simulink model "moresimilartoopenrocket"  (R2019a)
settings: Solver=ode4  StartTime=0.0  StopTime=6  FixedStep=0.0001  RelTol=1e-3
InitFcn:
  | HeightAboveSeaLevel = 5.4419142084;
  | Temperature = 288.15;
  | Pressure = 	101325;
  | 
  | GustStart = 2.5;
  | GustLength = [100, 100, 100];
  | GuestAmplitude = [ 2.5, -2.5,  1];
  | 
  | ShearSpeed = 10;
  | ShearDirection = 180;
values from neighbouring files (symbols this model uses):
  cg = temp(4)    [NonlinearStateEstimationForActuatorDelay.m]
  F = eye(6)    [MEKFAttitudeOnly.m]
  I = reshape(x(1:9), [3 3])    [AdaptiveLQR.m]    (also in MEKF.m = diag([0.08 0.08 0.002]); MEKFAttitudeOnly.m = diag([0.08 0.08 0.002]); MEKF_old.m = diag([0.08 0.08 0.002]); NonlinearStateEstimationForActuatorDelay.m = diag([Ixx, Ixx, Izz]))
  mass = 1.0565    [ImpactVelocityNotParallelMatlab.m]    (also in NonlinearStateEstimationForActuatorDelay.m = temp(1); OneDLanding.m; RunImpactVelocityParforCompiled.m; Tracker.m = 1.0616753546)
  q = x(13:16)    [AdaptiveLQR.m]    (also in MEKF.m = nominal_state(4:7); MEKFAttitudeOnly.m = [1 0 0 0]; MEKF_old.m = nominal_state(4:7); NonlinearStateEstimationForActuatorDelay.m = x(4:7))
  r = sym('r', [3 1])    [StateSpaceController.m]    (also in TimeDelayCompensationElevator.m = [0;0]; Tracker.m = [0; 0; -(rocket_length - Average_cg)])
undefined symbols (not defined in the file or in its folder): e0_0, e1_0, e2_0, e3_0, Earth, Light, MIL, WGS84
libraries: aerolibutil x5, aerolibwind2 x3, aerolibasang x2, simulink x2, aerolibatmos2 x1, aerolibbdyn x1, simulink_extras x1, aerolibtransform2 x1, sharedtransform x1
settings Model: Creator=rag  LastModifiedBy=rag

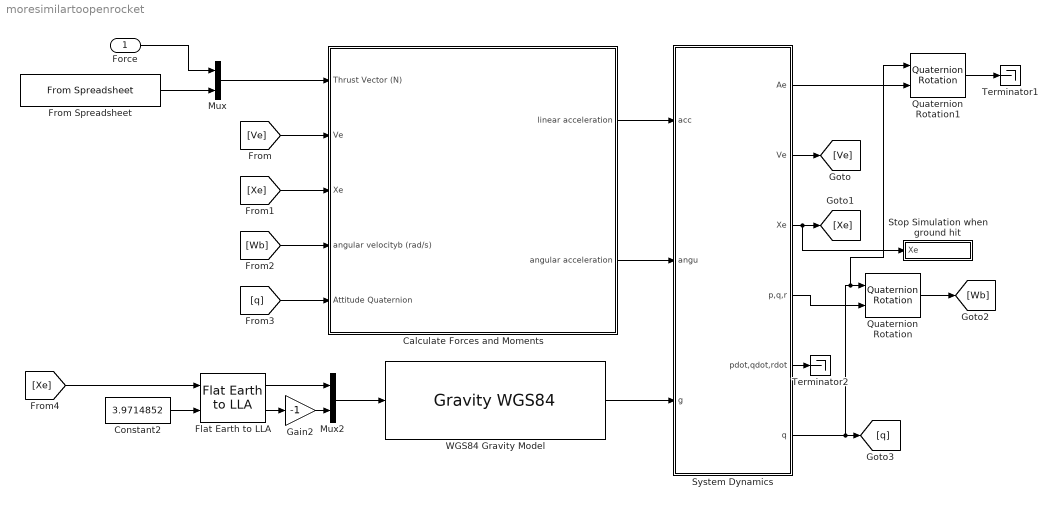
== system moresimilartoopenrocket ==
  Force : Inport  PortDimensions=2
  Calculate Forces and Moments : Subsystem
  Constant2 : Constant  Value=3.9714852
  Flat Earth to LLA : aerolibtransform2/Flat Earth to LLA  units=Metric (MKS)  ptype=Earth (WGS84)  F=1/298.257223563  R=6378137  LL0=[21.318358277648 -157.9232805920725]  psi=052
  From Spreadsheet : FromSpreadsheet  FileName=F10_Thrust.xls  ExtrapolationBeforeFirstDataPoint=Hold first value  ExtrapolationAfterLastDataPoint=Hold last value
  Gain2 : Gain  Gain=-1
  Mux : Mux  Inputs=2
  Mux2 : Mux  Inputs=2
  Quaternion Rotation : aerolibutil/Quaternion Rotation
  Quaternion Rotation1 : aerolibutil/Quaternion Rotation
  Stop Simulation when ground hit : Subsystem
  System Dynamics : Subsystem
  Terminator1 : Terminator
  Terminator2 : Terminator
  "WGS84 Gravity Model  " : GravityWGS84
  wires:
  Calculate Forces and Moments/2(angular acceleration) -> System Dynamics/2(angu)
  Mux/1 -> Calculate Forces and Moments/1(Thrust Vector (N))
  [Ve] -> Calculate Forces and Moments/2(Ve)
  [Xe] -> Calculate Forces and Moments/3(Xe)
  System Dynamics/3(Xe) -> Stop Simulation when ground hit/1(Xe), [Xe]
  Force/1 -> Mux/1
  From Spreadsheet/1 -> Mux/2
  Calculate Forces and Moments/1(linear acceleration) -> System Dynamics/1(acc)
  System Dynamics/2(Ve) -> [Ve]
  [Wb] -> Calculate Forces and Moments/4(angular velocityb (rad/s))
  [q] -> Calculate Forces and Moments/5(Attitude Quaternion)
  System Dynamics/5(pdot,qdot,rdot) -> Terminator2/1
  System Dynamics/6(q) -> [q], Quaternion Rotation1/1, Quaternion Rotation/1
  Constant2/1 -> Flat Earth to LLA/2
  [Xe] -> Flat Earth to LLA/1
  Flat Earth to LLA/1 -> Mux2/1
  Flat Earth to LLA/2 -> Gain2/1
  Mux2/1 -> "WGS84 Gravity Model  "/1
  Gain2/1 -> Mux2/2
  "WGS84 Gravity Model  "/1 -> System Dynamics/3(g)
  Quaternion Rotation/1 -> [Wb]
  System Dynamics/4(p,q,r) -> Quaternion Rotation/2
  Quaternion Rotation1/1 -> Terminator1/1
  System Dynamics/1(Ae) -> Quaternion Rotation1/2

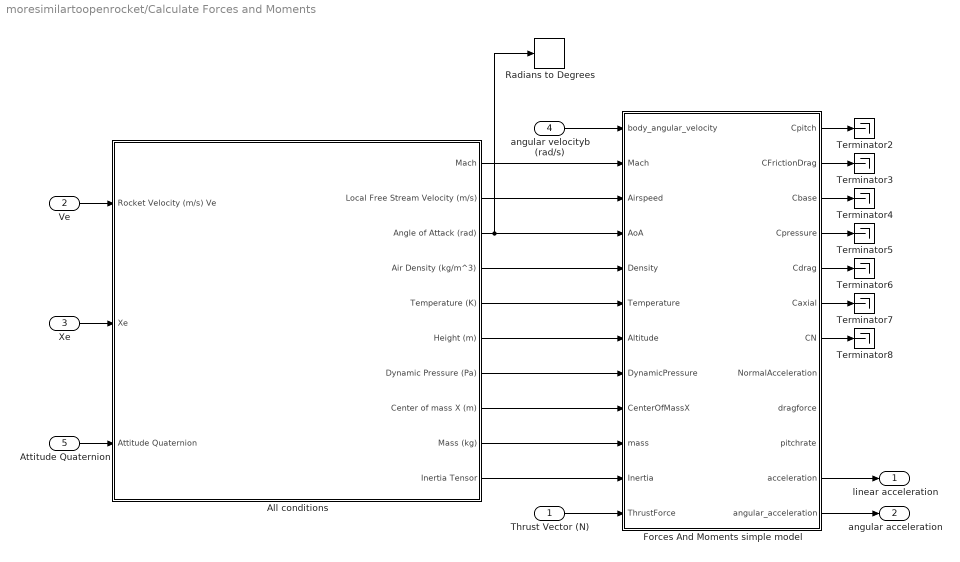
== system moresimilartoopenrocket/Calculate Forces and Moments ==
  Thrust Vector (N) : Inport
  Ve : Inport  Port=2
  Xe : Inport  Port=3
  angular velocityb (rad/s) : Inport  Port=4
  Attitude Quaternion : Inport  Port=5
  All conditions : Subsystem
  Forces And Moments simple model : MATLAB Function  TreatAsAtomicUnit=on
  Radians to Degrees : simulink_extras/Transformations/Radians to Degrees
  Terminator{2..8} (7 alike) : Terminator
  linear acceleration : Outport
  angular acceleration : Outport  Port=2
  wires:
  Forces And Moments simple model/4(Cpressure) -> Terminator5/1
  Xe/1 -> All conditions/2(Xe)
  Attitude Quaternion/1 -> All conditions/3(Attitude Quaternion)
  Forces And Moments simple model/1(Cpitch) -> Terminator2/1
  Forces And Moments simple model/3(Cbase) -> Terminator4/1
  Forces And Moments simple model/5(Cdrag) -> Terminator6/1
  Forces And Moments simple model/2(CFrictionDrag) -> Terminator3/1
  Forces And Moments simple model/6(Caxial) -> Terminator7/1
  Ve/1 -> All conditions/1(Rocket Velocity (m/s) Ve)
  Forces And Moments simple model/7(CN) -> Terminator8/1
  Forces And Moments simple model/12(angular_acceleration) -> angular acceleration/1
  Forces And Moments simple model/11(acceleration) -> linear acceleration/1
  All conditions/1(Mach) -> Forces And Moments simple model/2(Mach)
  All conditions/2(Local Free Stream Velocity (m/s)) -> Forces And Moments simple model/3(Airspeed)
  All conditions/4(Air Density (kg/m^3)) -> Forces And Moments simple model/5(Density)
  All conditions/3(Angle of Attack (rad)) -> Radians to Degrees/1, Forces And Moments simple model/4(AoA)
  All conditions/5(Temperature (K)) -> Forces And Moments simple model/6(Temperature)
  All conditions/7(Dynamic Pressure (Pa)) -> Forces And Moments simple model/8(DynamicPressure)
  All conditions/8(Center of mass X (m)) -> Forces And Moments simple model/9(CenterOfMassX)
  All conditions/6(Height (m)) -> Forces And Moments simple model/7(Altitude)
  All conditions/9(Mass (kg)) -> Forces And Moments simple model/10(mass)
  All conditions/10(Inertia Tensor) -> Forces And Moments simple model/11(Inertia)
  Thrust Vector (N)/1 -> Forces And Moments simple model/12(ThrustForce)
  angular velocityb (rad/s)/1 -> Forces And Moments simple model/1(body_angular_velocity)

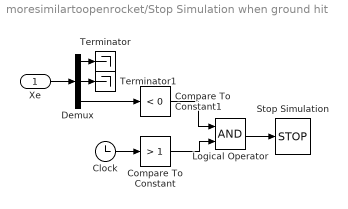
== system moresimilartoopenrocket/Stop Simulation when ground hit ==
  Xe : Inport
  Clock : Clock
  Compare To Constant : simulink/Logic and Bit Operations/Compare To Constant  relop=>  const=1  OutDataTypeStr=boolean
  Compare To Constant1 : simulink/Logic and Bit Operations/Compare To Constant  relop=<  const=0  OutDataTypeStr=boolean
  Demux : Demux  Outputs=3
  Logical Operator : Logic  AllPortsSameDT=off  OutDataTypeStr=boolean
  Stop Simulation : Stop
  Terminator : Terminator
  Terminator1 : Terminator
  wires:
  Logical Operator/1 -> Stop Simulation/1
  Compare To Constant/1 -> Logical Operator/2
  Clock/1 -> Compare To Constant/1
  Compare To Constant1/1 -> Logical Operator/1
  Xe/1 -> Demux/1
  Demux/1 -> Terminator/1
  Demux/2 -> Terminator1/1
  Demux/3 -> Compare To Constant1/1

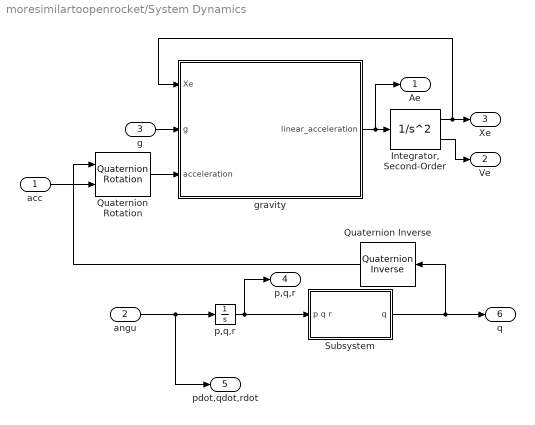
== system moresimilartoopenrocket/System Dynamics ==
  acc : Inport  Unit=N*m  PortDimensions=3
  angu : Inport  Port=2  PortDimensions=3
  g : Inport  Port=3
  "Integrator, Second-Order" : SecondOrderIntegrator
  Quaternion Inverse : aerolibutil/Quaternion Inverse
      settings: SourceProductName=Aerospace Blockset
  Quaternion Rotation : aerolibutil/Quaternion Rotation
  Subsystem : Subsystem
  gravity : MATLAB Function  TreatAsAtomicUnit=on
  "p,q,r " : Integrator
  Ae : Outport  Unit=m/s^2
  Ve : Outport  Port=2  Unit=m/s
  Xe : Outport  Port=3  Unit=m
  p,q,r : Outport  Port=4  Unit=rad/s
  pdot,qdot,rdot : Outport  Port=5  Unit=rad/s^2
  q : Outport  Port=6  Unit=1
  wires:
  "p,q,r "/1 -> p,q,r/1, Subsystem/1(p q r)
  angu/1 -> pdot,qdot,rdot/1, "p,q,r "/1
  acc/1 -> Quaternion Rotation/2
  Subsystem/1(q) -> Quaternion Inverse/1, q/1
  "Integrator, Second-Order"/1 -> Xe/1, gravity/1(Xe)
  "Integrator, Second-Order"/2 -> Ve/1
  Quaternion Rotation/1 -> gravity/3(acceleration)
  gravity/1(linear_acceleration) -> Ae/1, "Integrator, Second-Order"/1
  g/1 -> gravity/2(g)
  Quaternion Inverse/1 -> Quaternion Rotation/1

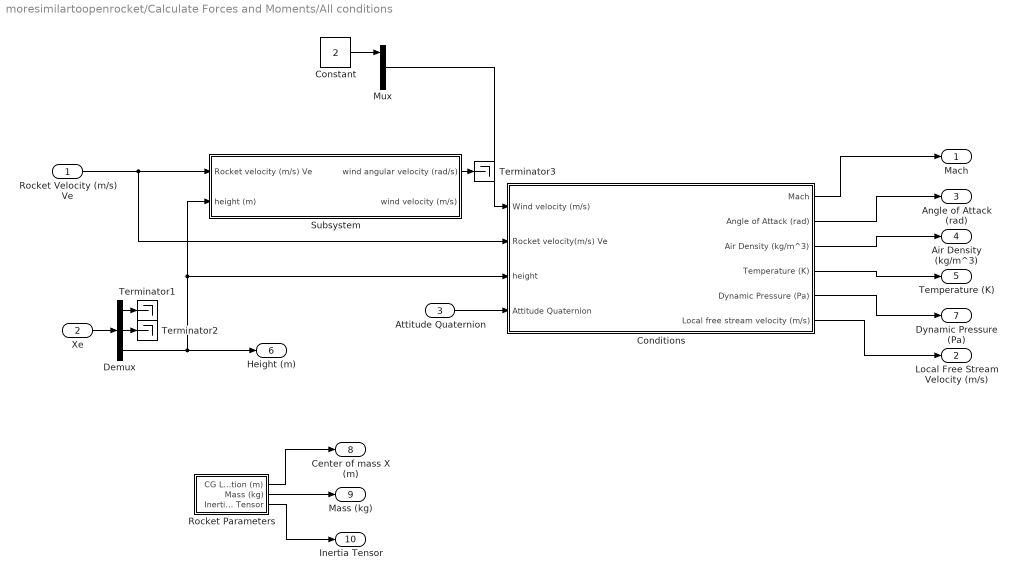
== system moresimilartoopenrocket/Calculate Forces and Moments/All conditions ==
  Rocket Velocity (m/s) Ve : Inport
  Xe : Inport  Port=2
  Attitude Quaternion : Inport  Port=3
  Conditions : Subsystem
  Constant : Constant  Value=2
  Demux : Demux  Outputs=3
  Mux : Mux  Inputs=3
  Rocket Parameters : Subsystem
  Subsystem : Subsystem
  Terminator1 : Terminator
  Terminator2 : Terminator
  Terminator3 : Terminator
  Mach : Outport
  Local Free Stream Velocity (m/s) : Outport  Port=2
  Angle of Attack (rad) : Outport  Port=3
  Air Density (kg/m^3) : Outport  Port=4
  Temperature (K) : Outport  Port=5
  Height (m) : Outport  Port=6
  Dynamic Pressure (Pa) : Outport  Port=7
  Center of mass X (m) : Outport  Port=8
  Mass (kg) : Outport  Port=9
  Inertia Tensor : Outport  Port=10
  wires:
  Demux/3 -> Height (m)/1, Conditions/3(height), Subsystem/2(height (m))
  Conditions/3(Air Density (kg/m^3)) -> Air Density (kg/m^3)/1
  Rocket Velocity (m/s) Ve/1 -> Subsystem/1(Rocket velocity (m/s) Ve), Conditions/2(Rocket velocity(m/s) Ve)
  Conditions/4(Temperature (K)) -> Temperature (K)/1
  Conditions/1(Mach) -> Mach/1
  Conditions/6(Local free stream velocity (m/s)) -> Local Free Stream Velocity (m/s)/1
  Demux/2 -> Terminator2/1
  Xe/1 -> Demux/1
  Rocket Parameters/1(CG Location (m)) -> Center of mass X (m)/1
  Rocket Parameters/3(Inertia Tensor) -> Inertia Tensor/1
  Conditions/2(Angle of Attack (rad)) -> Angle of Attack (rad)/1
  Demux/1 -> Terminator1/1
  Conditions/5(Dynamic Pressure (Pa)) -> Dynamic Pressure (Pa)/1
  Rocket Parameters/2(Mass (kg)) -> Mass (kg)/1
  Attitude Quaternion/1 -> Conditions/4(Attitude Quaternion)
  Mux/1 -> Conditions/1(Wind velocity (m/s))
  Constant/1 -> Mux/1
  Subsystem/1(wind angular velocity (rad/s)) -> Terminator3/1

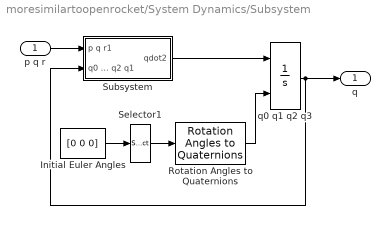
== system moresimilartoopenrocket/System Dynamics/Subsystem ==
  p q r : Inport
  Initial Euler Angles : Constant  Value=[0 0 0]
  Rotation Angles to Quaternions : sharedtransform/Rotation Angles to Quaternions  rotationOrder=ZYX  aMode=aMode
      settings: SourceProductName=Aerospace Blockset  SourceProductBaseCode=AE
  Selector1 : Selector  InputPortWidth=3  IndexOptions=Index vector (dialog)  Indices=[3 2 1]  OutputSizes=1
  Subsystem : Subsystem
  q0 q1 q2 q3 : Integrator  InitialConditionSource=external  InitialCondition=[e0_0 e1_0 e2_0 e3_0]
  q : Outport
  wires:
  Rotation Angles to Quaternions/1 -> q0 q1 q2 q3/2
  Initial Euler Angles/1 -> Selector1/1
  Subsystem/1(qdot2) -> q0 q1 q2 q3/1
  Selector1/1 -> Rotation Angles to Quaternions/1
  p q r/1 -> Subsystem/1(p q r1)
  q0 q1 q2 q3/1 -> q/1, Subsystem/2(q0 q1 q2 q1)

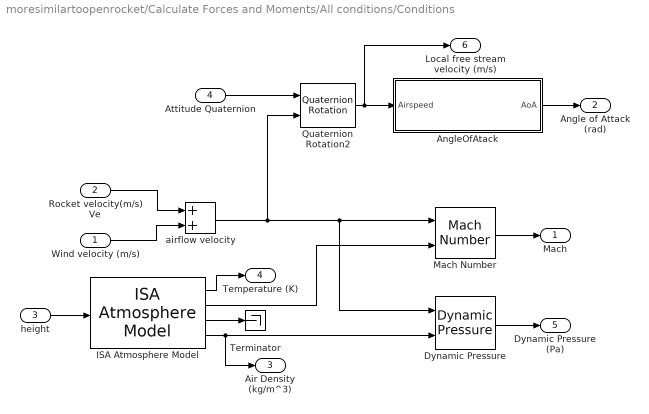
== system moresimilartoopenrocket/Calculate Forces and Moments/All conditions/Conditions ==
  Wind velocity (m/s) : Inport
  Rocket velocity(m/s) Ve : Inport  Port=2
  height : Inport  Port=3
  Attitude Quaternion : Inport  Port=4
  AngleOfAtack : MATLAB Function  TreatAsAtomicUnit=on
  Dynamic Pressure : aerolibasang/Dynamic Pressure
  ISA Atmosphere Model : aerolibatmos2/ISA Atmosphere Model  custom=on  g=9.80665  gamma=1.4  R=287.0531  L=0.0065  h_trop=11000  h_strat=20000  rho0=1.225  P0=Pressure  T0=Temperature  h0=0
      settings: SourceProductName=Aerospace Blockset
  Mach Number : aerolibasang/Mach Number
      settings: SourceProductName=Aerospace Blockset  SourceProductBaseCode=AE
  Quaternion Rotation2 : aerolibutil/Quaternion Rotation
  Terminator : Terminator
  airflow velocity : Sum
  Mach : Outport
  Angle of Attack (rad) : Outport  Port=2
  Air Density (kg/m^3) : Outport  Port=3
  Temperature (K) : Outport  Port=4
  Dynamic Pressure (Pa) : Outport  Port=5
  Local free stream velocity (m/s) : Outport  Port=6
  wires:
  ISA Atmosphere Model/4 -> Dynamic Pressure/2, Air Density (kg/m^3)/1
  ISA Atmosphere Model/2 -> Mach Number/2
  Dynamic Pressure/1 -> Dynamic Pressure (Pa)/1
  ISA Atmosphere Model/3 -> Terminator/1
  Mach Number/1 -> Mach/1
  Rocket velocity(m/s) Ve/1 -> airflow velocity/1
  ISA Atmosphere Model/1 -> Temperature (K)/1
  AngleOfAtack/1(AoA) -> Angle of Attack (rad)/1
  height/1 -> ISA Atmosphere Model/1
  Wind velocity (m/s)/1 -> airflow velocity/2
  Attitude Quaternion/1 -> Quaternion Rotation2/1
  airflow velocity/1 -> Quaternion Rotation2/2, Dynamic Pressure/1, Mach Number/1
  Quaternion Rotation2/1 -> AngleOfAtack/1(Airspeed), Local free stream velocity (m/s)/1

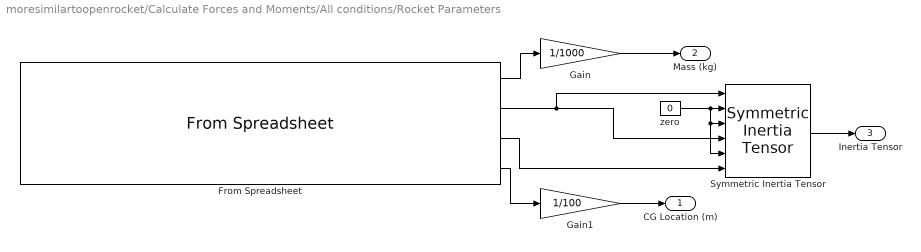
== system moresimilartoopenrocket/Calculate Forces and Moments/All conditions/Rocket Parameters ==
  From Spreadsheet : FromSpreadsheet  FileName=mass,cg,I.xlsx  SheetName=mass,cg,I  Range=A1:E251  ExtrapolationBeforeFirstDataPoint=Hold first value  ExtrapolationAfterLastDataPoint=Hold last value
  Gain : Gain  Gain=1/1000
  Gain1 : Gain  Gain=1/100
  Symmetric Inertia Tensor : aerolibbdyn/Symmetric Inertia Tensor
      settings: SourceProductName=Aerospace Blockset  SourceProductBaseCode=AE
  zero : Constant  Value=0
  CG Location (m) : Outport
  Mass (kg) : Outport  Port=2
  Inertia Tensor : Outport  Port=3
  wires:
  zero/1 -> Symmetric Inertia Tensor/5, Symmetric Inertia Tensor/3, Symmetric Inertia Tensor/2
  From Spreadsheet/2 -> Symmetric Inertia Tensor/1, Symmetric Inertia Tensor/4
  From Spreadsheet/3 -> Symmetric Inertia Tensor/6
  Symmetric Inertia Tensor/1 -> Inertia Tensor/1
  From Spreadsheet/4 -> Gain1/1
  From Spreadsheet/1 -> Gain/1
  Gain/1 -> Mass (kg)/1
  Gain1/1 -> CG Location (m)/1

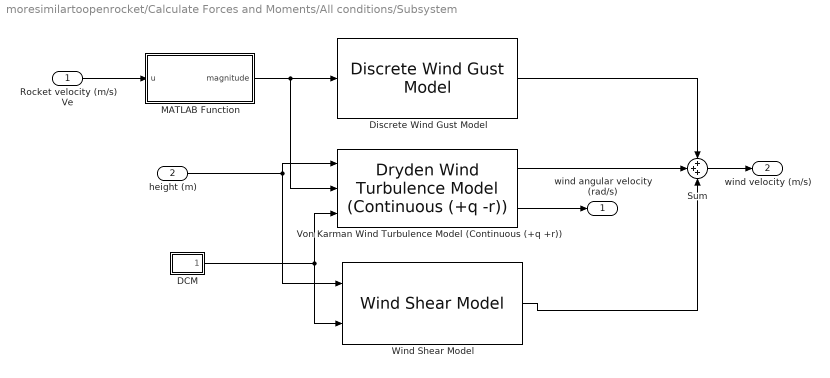
== system moresimilartoopenrocket/Calculate Forces and Moments/All conditions/Subsystem ==
  Rocket velocity (m/s) Ve : Inport
  height (m) : Inport  Port=2
  DCM : MATLAB Function  TreatAsAtomicUnit=on
  Discrete Wind Gust Model : aerolibwind2/Discrete Wind Gust Model  units=Metric (MKS)  Gx=on  Gy=on  Gz=on  t_0=GustStart  d_m=GustLength  v_m=GuestAmplitude
      settings: SourceProductName=Aerospace Blockset
  MATLAB Function : MATLAB Function  TreatAsAtomicUnit=on
  Sum : Sum  Inputs=3
  Von Karman Wind Turbulence Model (Continuous (+q +r)) : aerolibwind2/Dryden Wind Turbulence Model  (Continuous (+q -r))  units=Metric (MKS)  spec=MIL-F-8785C  model=Discrete Dryden (+q -r)  W20=ShearSpeed  Wdeg=ShearDirection  TurbProb=10^-2 - Light  L_high=762  Wingspan=10  ts=0.1  Seed=[23341 23342 23343 23344]  T_on=on
      settings: SourceProductName=Aerospace Blockset
  Wind Shear Model : aerolibwind2/Wind Shear Model  units=Metric (MKS)  phase=Category C - Terminal Flight Phase  W_20=ShearSpeed  Wdeg=ShearDirection
      settings: SourceProductName=Aerospace Blockset
  wind angular velocity (rad/s) : Outport
  wind velocity (m/s) : Outport  Port=2
  wires:
  height (m)/1 -> Wind Shear Model/1, Von Karman Wind Turbulence Model (Continuous (+q +r))/1
  Discrete Wind Gust Model/1 -> Sum/1
  DCM/1(DCM) -> Von Karman Wind Turbulence Model (Continuous (+q +r))/3, Wind Shear Model/2
  MATLAB Function/1(magnitude) -> Von Karman Wind Turbulence Model (Continuous (+q +r))/2, Discrete Wind Gust Model/1
  Sum/1 -> wind velocity (m/s)/1
  Wind Shear Model/1 -> Sum/3
  Von Karman Wind Turbulence Model (Continuous (+q +r))/1 -> Sum/2
  Von Karman Wind Turbulence Model (Continuous (+q +r))/2 -> wind angular velocity (rad/s)/1
  Rocket velocity (m/s) Ve/1 -> MATLAB Function/1(u)

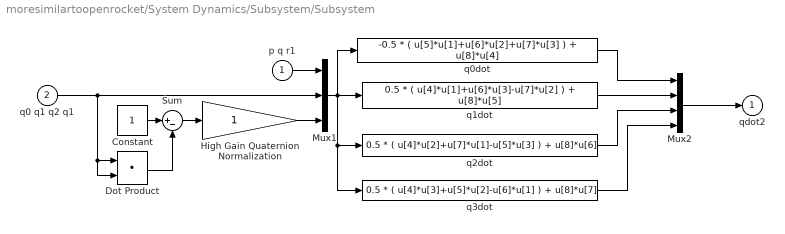
== system moresimilartoopenrocket/System Dynamics/Subsystem/Subsystem ==
  p q r1 : Inport
  q0 q1 q2 q1 : Inport  Port=2
  Constant : Constant
  Dot Product : DotProduct  OutDataTypeStr=Inherit: Inherit via internal rule
  High Gain Quaternion Normalization : Gain  SaturateOnIntegerOverflow=on  OutDataTypeStr=Inherit: Same as input  ParamDataTypeStr=Inherit: Same as input
  Mux1 : Mux  Inputs=[3 4 1]
  Mux2 : Mux
  Sum : Sum  Inputs=|+-  SaturateOnIntegerOverflow=on  InputSameDT=on  OutDataTypeStr=Inherit: Same as first input
  q0dot : Fcn  Expr=-0.5 * ( u[5]*u[1]+u[6]*u[2]+u[7]*u[3] ) + u[8]*u[4]
  q1dot : Fcn  Expr=0.5 * ( u[4]*u[1]+u[6]*u[3]-u[7]*u[2] ) + u[8]*u[5]
  q2dot : Fcn  Expr=0.5 * ( u[4]*u[2]+u[7]*u[1]-u[5]*u[3] ) + u[8]*u[6]
  q3dot : Fcn  Expr=0.5 * ( u[4]*u[3]+u[5]*u[2]-u[6]*u[1] ) + u[8]*u[7]
  qdot2 : Outport  InitialOutput=0
  wires:
  q0 q1 q2 q1/1 -> Dot Product/1, Dot Product/2, Mux1/2
  Mux1/1 -> q2dot/1, q3dot/1, q0dot/1, q1dot/1
  Constant/1 -> Sum/1
  High Gain Quaternion Normalization/1 -> Mux1/3
  q1dot/1 -> Mux2/2
  q0dot/1 -> Mux2/1
  Sum/1 -> High Gain Quaternion Normalization/1
  Dot Product/1 -> Sum/2
  q3dot/1 -> Mux2/4
  Mux2/1 -> qdot2/1
  q2dot/1 -> Mux2/3
  p q r1/1 -> Mux1/1

== matlab function moresimilartoopenrocket/Calculate Forces and Moments/Forces And Moments simple model ==
  settings: updateMethod=DISCRETE
  data: body_angular_velocity input; Mach input; Airspeed input size=[3 1]; AoA input; Density input; Temperature input; Altitude input; DynamicPressure input; CenterOfMassX input; mass input; Inertia input; Cpitch output; CFrictionDrag output; Cbase output; Cpressure output; Cdrag output; Caxial output; CN output; NormalAcceleration output; dragforce output; pitchrate output; acceleration output; angular_acceleration output; ThrustForce input
function [Cpitch, CFrictionDrag, Cbase, Cpressure, Cdrag, Caxial, CN, NormalAcceleration, dragforce, pitchrate, acceleration, angular_acceleration] = forces(body_angular_velocity, Mach, Airspeed, AoA, Density, Temperature, Altitude, DynamicPressure, CenterOfMassX, mass, Inertia, ThrustForce)
    persistent ThetaRotation
    if isempty(ThetaRotation)
         ThetaRotation = eye(3);
    end

    %% Rocket Shape Constants
    Reference_Diameter = 7.62e-2;
    Reference_Radius = Reference_Diameter / 2;
    Reference_Area = Reference_Radius^2 * pi;
    
    NoseCone_Length = 15e-2;
    BodyTube_Length = 80e-2; 
    NoseCone_WetArea = pi * Reference_Radius * NoseCone_Length;          % pi*r*l 
    BodyTube_WetArea = pi * Reference_Radius * 2 * BodyTube_Length;      % pi*d*l
    NoseCone_PlanformArea = Reference_Diameter * NoseCone_Length / 2;
    BodyTube_PlanformArea = Reference_Diameter * BodyTube_Length;
    
    SurfaceRoughness = 20e-6;
    
    sinphi = Reference_Radius / hypot(Reference_Radius, NoseCone_Length);
    BodyTube_CP = 0.55;
    NoseCone_CP = 0.1;
    PitchCenterX = 0;
   
    
    COT_to_COM = .95 - CenterOfMassX; %get actual value and change over time as solid motor burns
    
    %% General Constants
    K = 1.1;
   
    %% Coefficients
    pitchrate = ThetaRotation \ body_angular_velocity;
    [CN, Cpitch] = CalculatePitchAndNormalCDs(Mach, K, Reference_Diameter, AoA, Airspeed, pitchrate(2), NoseCone_Length, BodyTube_Length, Reference_Area, CenterOfMassX, PitchCenterX, NoseCone_PlanformArea, BodyTube_PlanformArea, NoseCone_CP, BodyTube_CP);
    
    Cbase = .12 + .13*Mach^2;
    CFrictionDrag = CalculateFrictionDrag(Temperature, Density, Reference_Radius, Reference_Area, SurfaceRoughness, NoseCone_Length, BodyTube_Length, Airspeed, Mach, NoseCone_WetArea, BodyTube_WetArea);
    Cpressure = PressureDragForce(sinphi);
    
    Cdrag = Cbase + CFrictionDrag + Cpressure;
    Caxial = AxialDragMul(AoA) * Cdrag;
    
    Cyaw = 0.0;
    
    Croll = 0.0;
    Cside = 0;
    
    %% Forces and Moments
    z = DynamicPressure * Reference_Area;
    
    lengtha = norm(Airspeed(1:2));
    
    sina = Airspeed(2) / lengtha;
    cosa = Airspeed(1) / lengtha;

    ThetaRotation = [cosa, -sina, 0; sina, cosa, 0; 0, 0, 1];
    %ThetaRotation = rotz(acos(Airspeed(1)/lengtha));
    
    Thrust_moment = COT_to_COM * [ThrustForce(2); ThrustForce(1); 0];
    
    dragforce = z * Caxial;
    NormalAcceleration = z * -CN / mass;
    
    acceleration = (z * -[CN; Cside; Caxial] + ThrustForce) / mass; 
    acceleration = ThetaRotation * acceleration;
    angular_acceleration = z * Reference_Diameter * [-Cyaw / Inertia(1,1); Cpitch / Inertia(1,1) ; Croll/ Inertia(3,3)];
    angular_acceleration = ThetaRotation * angular_acceleration + Thrust_moment;
    
    if Altitude <= 0
        acceleration = [0;0;acceleration(3)];
        angular_acceleration = [0; 0; 0];
    end

end

== matlab function moresimilartoopenrocket/System Dynamics/gravity ==
  settings: updateMethod=DISCRETE
  data: Xe input; g input; linear_acceleration output; acceleration input
function linear_acceleration = addgravity(Xe, g, acceleration)
    linear_acceleration = acceleration - g;
    
    if linear_acceleration(3) < 0 && Xe(3) <= 0
        linear_acceleration(3) = 0;
        
    end

== matlab function moresimilartoopenrocket/Calculate Forces and Moments/All conditions/Conditions/AngleOfAtack ==
  settings: updateMethod=DISCRETE
  data: Airspeed input; AoA output
function AoA = AngleOfAttack(Airspeed)
    AoA = acos(Airspeed(3) / norm(Airspeed));
        
    if norm(Airspeed) <= .01
        AoA = 0;
    end
end

== matlab function moresimilartoopenrocket/Calculate Forces and Moments/All conditions/Subsystem/DCM ==
  settings: updateMethod=DISCRETE
  data: DCM output
function DCM  = forces
    DCM = [1,0,0;0,1,0;0,0,1];

== matlab function moresimilartoopenrocket/Calculate Forces and Moments/All conditions/Subsystem/MATLAB Function ==
  data: u input; magnitude output
function magnitude = VectorNorm(u)
    magnitude = norm(u);
